simulink model "pb_model"  (R2019b)
settings: Solver=ode45  StartTime=0.0  StopTime=sim_time  FixedStep=0.025  MaxStep=0.025  RelTol=1e-4  AbsTol=1e-4
values from neighbouring files (symbols this model uses):
  A = matrix_A(theta)    [PENDUBOT.m]    (also in matrix_A.m = [0, 1, 0, 0;       -(theta(6)*(theta(2)*theta(4) - theta(3)*; pendubot_animation.m = [A0; A1; A2; A3; A4; A5; A0])
  B = matrix_B(theta)    [PENDUBOT.m]    (also in matrix_B.m = [0;       theta(2)/(- theta(3)^2 + theta(1)*theta(2));      ; pendubot_animation.m = [B0; B1; B2; B3; B4; B5; B0])
  C = [1 0 0 0;       0 0 1 0]    [PENDUBOT.m]
  L = L_    [finding_l0.m]    (also in pole_del.m = [])
  theta = [0.014680882,0.00223765,0.00146916,0.060038,0.00693,9.81,0.0001,0.0001]    [PENDUBOT.m]    (also in phis_param2theta.m = [m1*lc1^2 + m2*l1^2 + I1, m2*lc2^2 + I2, m2*l1*lc2, m1*lc1 +)
  X0 = [pi/4; 0; 0; 0]    [PENDUBOT.m]    (also in lipschitz_const_check.m = zeros(2,3))
  Z0 = [pi/2; 0; 0; 0]    [PENDUBOT.m]
undefined symbols (not defined in the file or in its folder): K_mid, K_up, lips_func, observ_func, pendubot_control
settings Model: Creator=thrus  LastModifiedBy=thrus
settings SolverCC: AutoScaleAbsTol=off
settings DataIOCC: ReturnWorkspaceOutputs=off
settings DebuggingCC: ArithmeticOperatorsInVariantConditions=warning
settings SFSimCC: SimUseLocalCustomCode=off  CustomCodeUndefinedFunction=UseInterfaceOnly
settings RTWCC: RTWUseLocalCustomCode=off

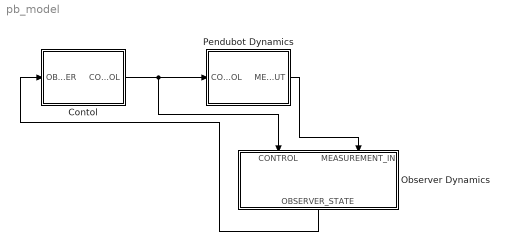
== system pb_model ==
  Contol : Subsystem
      mask Display: disp('CONTROL')
  Observer Dynamics : Subsystem
      mask Display: disp('ASYMPTOTIC\nOBSERVER')
  Pendubot Dynamics : Subsystem
      mask Display: disp('PENDUBOT')
  wires:
  Pendubot Dynamics/1(MEASUREMENT_OUT) -> Observer Dynamics/2(MEASUREMENT_IN)
  Observer Dynamics/1(OBSERVER_STATE) -> Contol/1(OBSERVER)
  Contol/1(CONTROL) -> Observer Dynamics/1(CONTROL), Pendubot Dynamics/1(CONTROL)

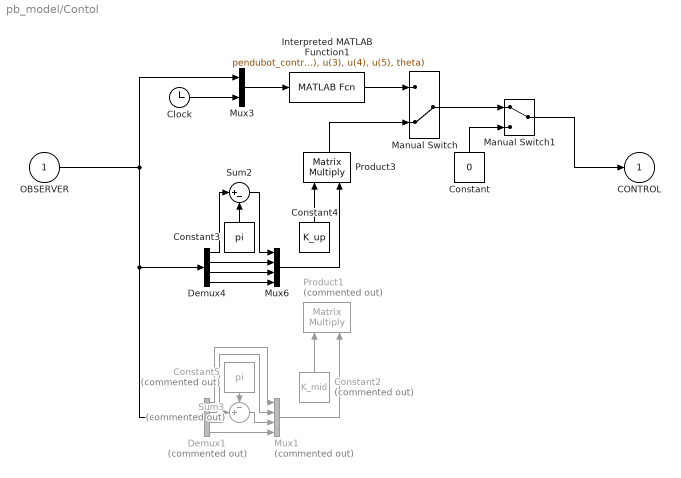
== system pb_model/Contol ==
  OBSERVER : Inport
  Clock : Clock
  Constant : Constant  Value=0
  Constant2 : Constant  Commented=on  Value=K_mid  VectorParams1D=off
  Constant3 : Constant  Value=pi  VectorParams1D=off
  Constant4 : Constant  Value=K_up  VectorParams1D=off
  Constant5 : Constant  Commented=on  Value=pi  VectorParams1D=off
  Demux1 : Demux  Commented=on
  Demux4 : Demux
  Interpreted MATLAB Function1 : MATLABFcn  MATLABFcn=pendubot_control(u(1), u(2), u(3), u(4), u(5), theta)  OutputDimensions=1
      mask Display: disp('Control')
  Manual Switch : ManualSwitch  CurrentSetting=0
  Manual Switch1 : ManualSwitch
  Mux1 : Mux  Commented=on
  Mux3 : Mux  Inputs=2
  Mux6 : Mux
  Product1 : Product  Commented=on  Multiplication=Matrix(*)
  Product3 : Product  Multiplication=Matrix(*)
  Sum2 : Sum  Inputs=|+-
  Sum3 : Sum  Commented=on  Inputs=-+|
  CONTROL : Outport
  wires:
  Demux4/1 -> Sum2/1
  Mux6/1 -> Product3/2
  Constant3/1 -> Sum2/2
  Demux4/4 -> Mux6/4
  Sum2/1 -> Mux6/1
  Demux4/3 -> Mux6/3
  Clock/1 -> Mux3/2
  Mux3/1 -> Interpreted MATLAB Function1/1
  Demux4/2 -> Mux6/2
  Constant4/1 -> Product3/1
  Interpreted MATLAB Function1/1 -> Manual Switch/1
  Manual Switch/1 -> Manual Switch1/1
  Constant/1 -> Manual Switch1/2
  Manual Switch1/1 -> CONTROL/1
  Constant2/1 -> Product1/1
  OBSERVER/1 -> Mux3/1, Demux1/1, Demux4/1
  Mux1/1 -> Product1/2
  Demux1/2 -> Mux1/2
  Demux1/3 -> Sum3/2
  Sum3/1 -> Mux1/3
  Constant5/1 -> Sum3/1
  Demux1/4 -> Mux1/4
  Demux1/1 -> Mux1/1
  Product3/1 -> Manual Switch/2

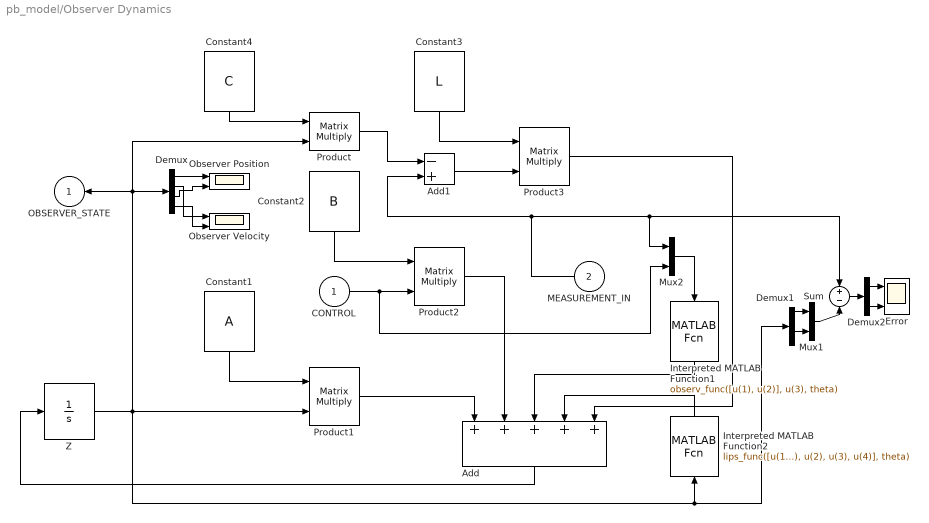
== system pb_model/Observer Dynamics ==
  CONTROL : Inport
  MEASUREMENT_IN : Inport  Port=2
  Add : Sum  Inputs=+++++
  Add1 : Sum  Inputs=-+
  Constant1 : Constant  Value=A  VectorParams1D=off
  Constant2 : Constant  Value=B  VectorParams1D=off
  Constant3 : Constant  Value=L  VectorParams1D=off
  Constant4 : Constant  Value=C  VectorParams1D=off
  Demux : Demux
  Demux1 : Demux
  Demux2 : Demux  Outputs=2
  Error : Scope  NumInputPorts=2
  Interpreted MATLAB Function1 : MATLABFcn  MATLABFcn=observ_func([u(1), u(2)], u(3), theta)  OutputDimensions=4  Output1D=off
      mask Display: disp('f(t, u, y)')
  Interpreted MATLAB Function2 : MATLABFcn  MATLABFcn=lips_func([u(1), u(2), u(3), u(4)], theta)  OutputDimensions=4  Output1D=off
      mask Display: disp('g(t, u, x)')
  Mux1 : Mux  Inputs=2
  Mux2 : Mux  Inputs=2
  Observer Position : Scope  NumInputPorts=2
  Observer Velocity : Scope  NumInputPorts=2
  Product{,1..3} (4 alike) : Product  Multiplication=Matrix(*)
  Sum : Sum  Inputs=+-
  Z : Integrator  InitialCondition=Z0
  OBSERVER_STATE : Outport
  wires:
  Demux/3 -> Observer Position/2
  Demux/1 -> Observer Position/1
  Demux/4 -> Observer Velocity/2
  Demux/2 -> Observer Velocity/1
  Demux1/1 -> Mux1/1
  Demux1/3 -> Mux1/2
  Mux1/1 -> Sum/2
  Sum/1 -> Demux2/1
  Demux2/1 -> Error/1
  Demux2/2 -> Error/2
  Add/1 -> Z/1
  Constant2/1 -> Product2/1
  Constant1/1 -> Product1/1
  Interpreted MATLAB Function2/1 -> Add/4
  Interpreted MATLAB Function1/1 -> Add/3
  Mux2/1 -> Interpreted MATLAB Function1/1
  Product1/1 -> Add/1
  Product2/1 -> Add/2
  CONTROL/1 -> Product2/2, Mux2/2
  Constant3/1 -> Product3/1
  Add1/1 -> Product3/2
  MEASUREMENT_IN/1 -> Add1/2, Sum/1, Mux2/1
  Z/1 -> Product1/2, OBSERVER_STATE/1, Product/2, Demux/1, Interpreted MATLAB Function2/1, Demux1/1
  Constant4/1 -> Product/1
  Product/1 -> Add1/1
  Product3/1 -> Add/5

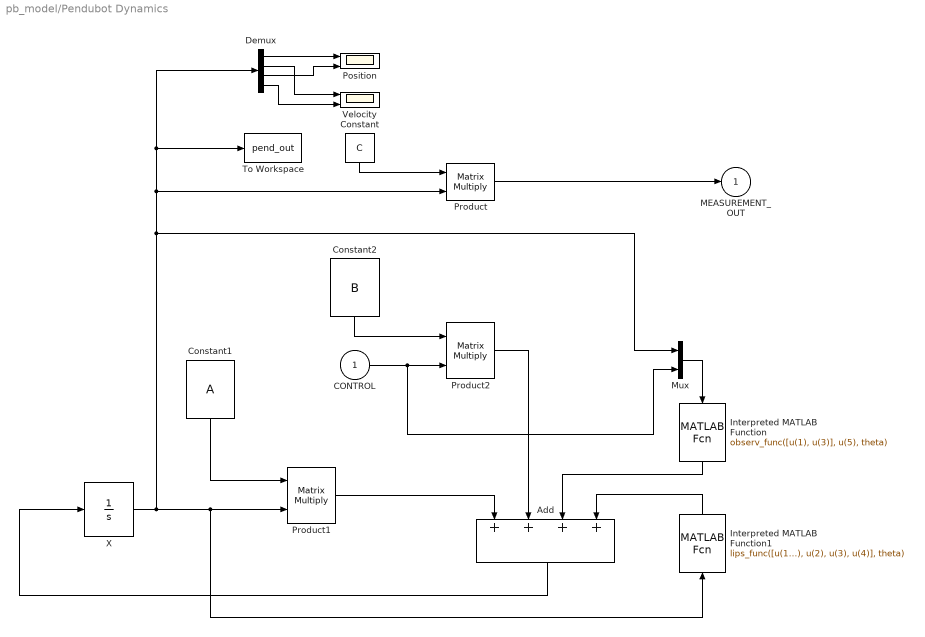
== system pb_model/Pendubot Dynamics ==
  CONTROL : Inport
  Add : Sum  Inputs=++++
  Constant : Constant  Value=C  VectorParams1D=off
  Constant1 : Constant  Value=A  VectorParams1D=off
  Constant2 : Constant  Value=B  VectorParams1D=off
  Demux : Demux
  Interpreted MATLAB Function : MATLABFcn  MATLABFcn=observ_func([u(1), u(3)], u(5), theta)  OutputDimensions=4  Output1D=off
      mask Display: disp('f(t, u, y)')
  Interpreted MATLAB Function1 : MATLABFcn  MATLABFcn=lips_func([u(1), u(2), u(3), u(4)], theta)  OutputDimensions=4  Output1D=off
      mask Display: disp('g(t, u, x)')
  Mux : Mux  Inputs=2
  Position : Scope  NumInputPorts=2
  Product : Product  Multiplication=Matrix(*)
  Product1 : Product  Multiplication=Matrix(*)
  Product2 : Product  Multiplication=Matrix(*)
  To Workspace : ToWorkspace  VariableName=pend_out  SaveFormat=Structure With Time  SampleTime=-1
  Velocity : Scope  NumInputPorts=2
  X : Integrator  InitialCondition=X0
  MEASUREMENT_OUT : Outport
  wires:
  Product/1 -> MEASUREMENT_OUT/1
  Constant/1 -> Product/1
  Demux/3 -> Position/2
  Demux/1 -> Position/1
  Demux/4 -> Velocity/2
  Demux/2 -> Velocity/1
  Constant2/1 -> Product2/1
  Add/1 -> X/1
  X/1 -> Product/2, To Workspace/1, Demux/1, Mux/1, Product1/2, Interpreted MATLAB Function1/1
  Product2/1 -> Add/2
  CONTROL/1 -> Product2/2, Mux/2
  Mux/1 -> Interpreted MATLAB Function/1
  Interpreted MATLAB Function/1 -> Add/3
  Interpreted MATLAB Function1/1 -> Add/4
  Product1/1 -> Add/1
  Constant1/1 -> Product1/1
